simulink model "Assignment8"  (R2017a)
settings: Solver=FixedStepAuto  StartTime=0.0  StopTime=10.0  FixedStep=1e-5  RelTol=1e-3
values from neighbouring files (symbols this model uses):
  B = 0.1    [Assignment8_case1.m]    (also in Assignment8_case2.m; Assignment8_case3.m; Assignment8_case4.m; Assignment8_case5.m)
  FV = 10    [Assignment8_case1.m]    (also in Assignment8_case2.m = 900; Assignment8_case3.m; Assignment8_case4.m; Assignment8_case5.m)
  J = 0.01    [Assignment8_case1.m]    (also in Assignment8_case2.m; Assignment8_case3.m; Assignment8_case4.m; Assignment8_case5.m)
  K = 0.1    [Assignment8_case1.m]    (also in Assignment8_case2.m; Assignment8_case3.m; Assignment8_case4.m; Assignment8_case5.m)
  La = 0.5e-3    (= 0.0005)    [Assignment8_case1.m]    (also in Assignment8_case2.m; Assignment8_case3.m; Assignment8_case4.m; Assignment8_case5.m)
  Ra = 10    [Assignment8_case1.m]    (also in Assignment8_case2.m; Assignment8_case3.m; Assignment8_case4.m; Assignment8_case5.m)
  Step = 0    [Assignment8_case1.m]    (also in Assignment8_case2.m; Assignment8_case3.m; Assignment8_case4.m; Assignment8_case5.m)
settings Model: Creator=jms2299  LastModifiedBy=jms2299

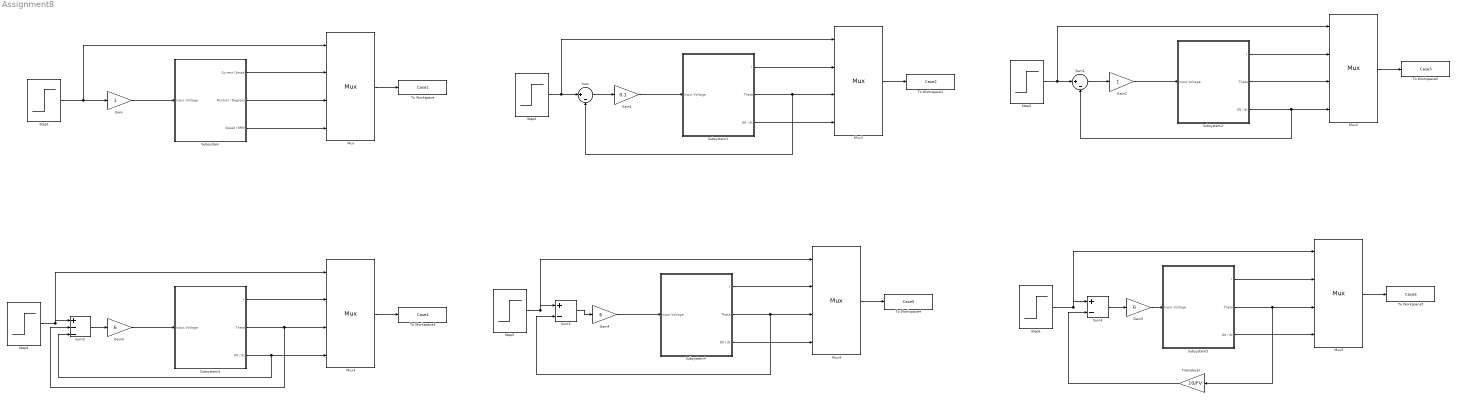
== system Assignment8 ==
  Gain : Gain
  Gain1 : Gain  Gain=0.1
  Gain2 : Gain
  Gain3 : Gain  Gain=6
  Gain4 : Gain  Gain=6
  Gain5 : Gain  Gain=6
  Mux{,1..5} (6 alike) : Mux
  Step{1..6} (6 alike) : Step  Time=Step  After=FV  SampleTime=0
  Subsystem : Subsystem
  Subsystem1 : Subsystem
  Subsystem2 : Subsystem
  Subsystem3 : Subsystem
  Subsystem4 : Subsystem
  Subsystem5 : Subsystem
  Sum{,1,3..4} (4 alike) : Sum  Inputs=|+-
  Sum2 : Sum  Inputs=|+--
  To Workspace : ToWorkspace  VariableName=Case1  SampleTime=-1
  To Workspace1 : ToWorkspace  VariableName=Case2  SampleTime=-1
  To Workspace2 : ToWorkspace  VariableName=Case3  SampleTime=-1
  To Workspace3 : ToWorkspace  VariableName=Case4  SampleTime=-1
  To Workspace4 : ToWorkspace  VariableName=Case5  SampleTime=-1
  To Workspace5 : ToWorkspace  VariableName=Case6  SampleTime=-1
  Transducer : Gain  Gain=10/FV
  wires:
  Step1/1 -> Mux/1, Gain/1
  Subsystem/2(Position (Degrees)) -> Mux/3
  Subsystem/1(Current (Amps)) -> Mux/2
  Subsystem/3(Speed (RPM)) -> Mux/4
  Mux/1 -> To Workspace/1
  Gain/1 -> Subsystem/1(Input Voltage)
  Mux1/1 -> To Workspace1/1
  Gain1/1 -> Subsystem1/1(Input Voltage)
  Subsystem1/3(D0 / dt) -> Mux1/4
  Subsystem1/1(I) -> Mux1/2
  Sum/1 -> Gain1/1
  Step2/1 -> Mux1/1, Sum/1
  Subsystem1/2(Theta) -> Sum/2, Mux1/3
  Step3/1 -> Mux2/1, Sum1/1
  Subsystem2/3(D0 / dt) -> Sum1/2, Mux2/4
  Subsystem2/2(Theta) -> Mux2/3
  Subsystem2/1(I) -> Mux2/2
  Gain2/1 -> Subsystem2/1(Input Voltage)
  Sum1/1 -> Gain2/1
  Mux2/1 -> To Workspace2/1
  Step4/1 -> Mux3/1, Sum2/1
  Subsystem3/3(D0 / dt) -> Sum2/3, Mux3/4
  Subsystem3/2(Theta) -> Sum2/2, Mux3/3
  Subsystem3/1(I) -> Mux3/2
  Gain3/1 -> Subsystem3/1(Input Voltage)
  Sum2/1 -> Gain3/1
  Mux3/1 -> To Workspace3/1
  Mux4/1 -> To Workspace4/1
  Subsystem4/2(Theta) -> Sum3/2, Mux4/3
  Subsystem4/1(I) -> Mux4/2
  Step5/1 -> Mux4/1, Sum3/1
  Subsystem4/3(D0 / dt) -> Mux4/4
  Sum3/1 -> Gain4/1
  Gain4/1 -> Subsystem4/1(Input Voltage)
  Subsystem5/3(D0 / dt) -> Mux5/4
  Subsystem5/2(Theta) -> Transducer/1, Mux5/3
  Subsystem5/1(I) -> Mux5/2
  Mux5/1 -> To Workspace5/1
  Transducer/1 -> Sum4/2
  Step6/1 -> Mux5/1, Sum4/1
  Sum4/1 -> Gain5/1
  Gain5/1 -> Subsystem5/1(Input Voltage)

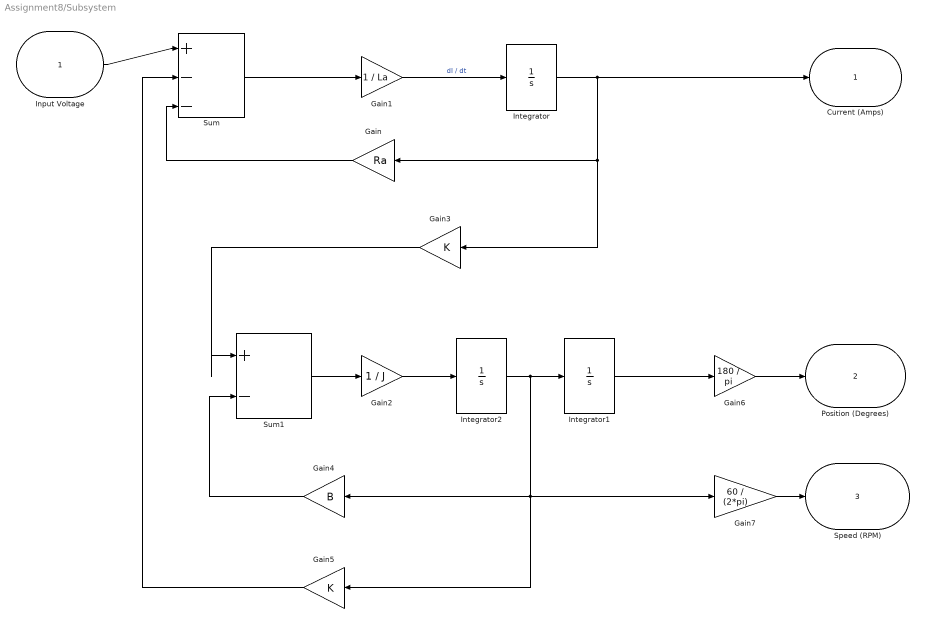
== system Assignment8/Subsystem ==
  Input Voltage : Inport
  Gain : Gain  Gain=Ra
  Gain1 : Gain  Gain=1 / La
  Gain2 : Gain  Gain=1 / J
  Gain3 : Gain  Gain=K
  Gain4 : Gain  Gain=B
  Gain5 : Gain  Gain=K
  Gain6 : Gain  Gain=180 / pi
  Gain7 : Gain  Gain=60 / (2*pi)
  Integrator : Integrator
  Integrator1 : Integrator
  Integrator2 : Integrator
  Sum : Sum  Inputs=|+--
  Sum1 : Sum  Inputs=|+-
  Current (Amps) : Outport
  Position (Degrees) : Outport  Port=2
  Speed (RPM) : Outport  Port=3
  wires:
  Sum1/1 -> Gain2/1
  Integrator/1 -> Current (Amps)/1, Gain3/1, Gain/1
  Gain3/1 -> Sum1/1
  Gain/1 -> Sum/3
  Gain1/1 -> Integrator/1  "dI / dt"
  Gain2/1 -> Integrator2/1
  Sum/1 -> Gain1/1
  Gain4/1 -> Sum1/2
  Gain5/1 -> Sum/2
  Integrator2/1 -> Gain7/1, Gain4/1, Gain5/1, Integrator1/1
  Input Voltage/1 -> Sum/1
  Integrator1/1 -> Gain6/1
  Gain6/1 -> Position (Degrees)/1
  Gain7/1 -> Speed (RPM)/1

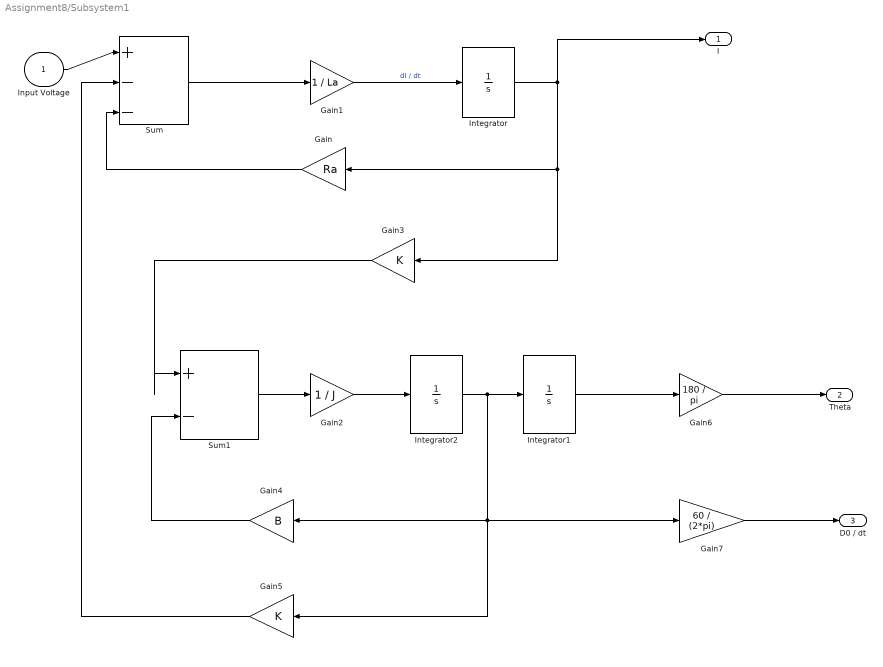
== system Assignment8/Subsystem1 ==
  Input Voltage : Inport
  Gain : Gain  Gain=Ra
  Gain1 : Gain  Gain=1 / La
  Gain2 : Gain  Gain=1 / J
  Gain3 : Gain  Gain=K
  Gain4 : Gain  Gain=B
  Gain5 : Gain  Gain=K
  Gain6 : Gain  Gain=180 / pi
  Gain7 : Gain  Gain=60 / (2*pi)
  Integrator : Integrator
  Integrator1 : Integrator
  Integrator2 : Integrator
  Sum : Sum  Inputs=|+--
  Sum1 : Sum  Inputs=|+-
  I : Outport
  Theta : Outport  Port=2
  D0 / dt : Outport  Port=3
  wires:
  Sum1/1 -> Gain2/1
  Integrator/1 -> I/1, Gain3/1, Gain/1
  Gain3/1 -> Sum1/1
  Gain/1 -> Sum/3
  Gain1/1 -> Integrator/1  "dI / dt"
  Gain2/1 -> Integrator2/1
  Sum/1 -> Gain1/1
  Gain4/1 -> Sum1/2
  Gain5/1 -> Sum/2
  Integrator2/1 -> Gain7/1, Gain4/1, Gain5/1, Integrator1/1
  Input Voltage/1 -> Sum/1
  Integrator1/1 -> Gain6/1
  Gain6/1 -> Theta/1
  Gain7/1 -> D0 / dt/1

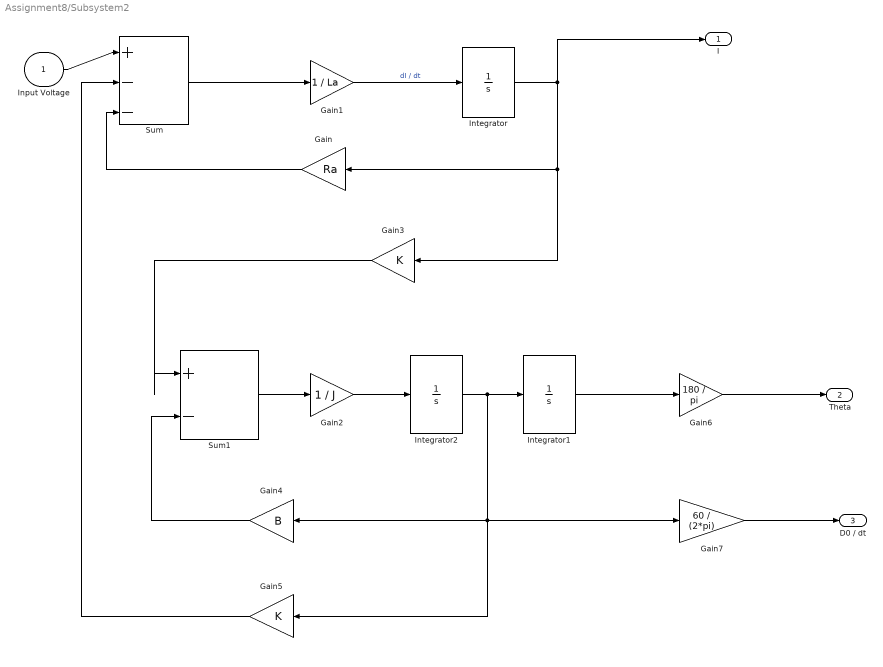
== system Assignment8/Subsystem2 ==
  Input Voltage : Inport
  Gain : Gain  Gain=Ra
  Gain1 : Gain  Gain=1 / La
  Gain2 : Gain  Gain=1 / J
  Gain3 : Gain  Gain=K
  Gain4 : Gain  Gain=B
  Gain5 : Gain  Gain=K
  Gain6 : Gain  Gain=180 / pi
  Gain7 : Gain  Gain=60 / (2*pi)
  Integrator : Integrator
  Integrator1 : Integrator
  Integrator2 : Integrator
  Sum : Sum  Inputs=|+--
  Sum1 : Sum  Inputs=|+-
  I : Outport
  Theta : Outport  Port=2
  D0 / dt : Outport  Port=3
  wires:
  Sum1/1 -> Gain2/1
  Integrator/1 -> I/1, Gain3/1, Gain/1
  Gain3/1 -> Sum1/1
  Gain/1 -> Sum/3
  Gain1/1 -> Integrator/1  "dI / dt"
  Gain2/1 -> Integrator2/1
  Sum/1 -> Gain1/1
  Gain4/1 -> Sum1/2
  Gain5/1 -> Sum/2
  Integrator2/1 -> Gain7/1, Gain4/1, Gain5/1, Integrator1/1
  Input Voltage/1 -> Sum/1
  Integrator1/1 -> Gain6/1
  Gain6/1 -> Theta/1
  Gain7/1 -> D0 / dt/1

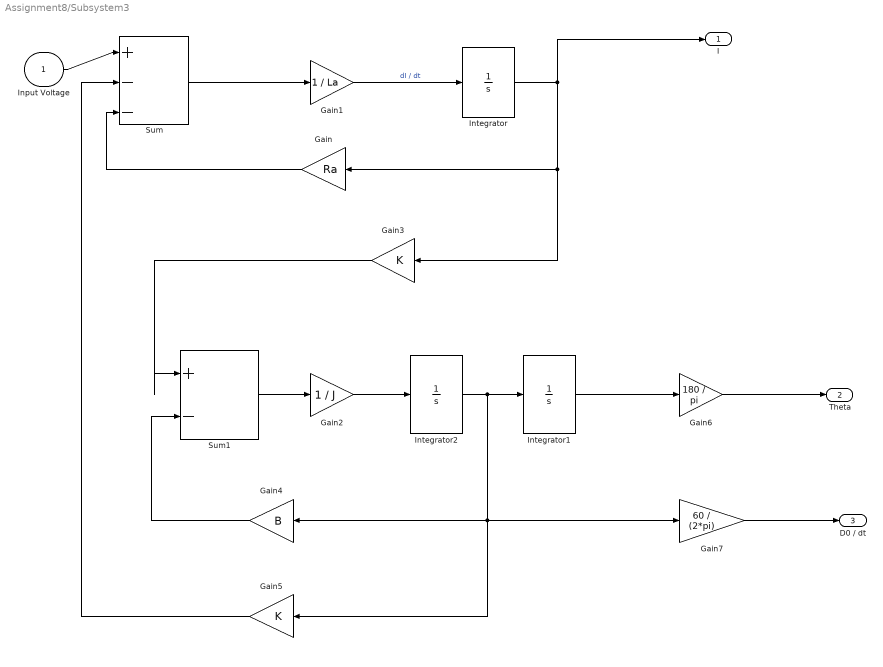
== system Assignment8/Subsystem3 ==
  Input Voltage : Inport
  Gain : Gain  Gain=Ra
  Gain1 : Gain  Gain=1 / La
  Gain2 : Gain  Gain=1 / J
  Gain3 : Gain  Gain=K
  Gain4 : Gain  Gain=B
  Gain5 : Gain  Gain=K
  Gain6 : Gain  Gain=180 / pi
  Gain7 : Gain  Gain=60 / (2*pi)
  Integrator : Integrator
  Integrator1 : Integrator
  Integrator2 : Integrator
  Sum : Sum  Inputs=|+--
  Sum1 : Sum  Inputs=|+-
  I : Outport
  Theta : Outport  Port=2
  D0 / dt : Outport  Port=3
  wires:
  Sum1/1 -> Gain2/1
  Integrator/1 -> I/1, Gain3/1, Gain/1
  Gain3/1 -> Sum1/1
  Gain/1 -> Sum/3
  Gain1/1 -> Integrator/1  "dI / dt"
  Gain2/1 -> Integrator2/1
  Sum/1 -> Gain1/1
  Gain4/1 -> Sum1/2
  Gain5/1 -> Sum/2
  Integrator2/1 -> Gain7/1, Gain4/1, Gain5/1, Integrator1/1
  Input Voltage/1 -> Sum/1
  Integrator1/1 -> Gain6/1
  Gain6/1 -> Theta/1
  Gain7/1 -> D0 / dt/1

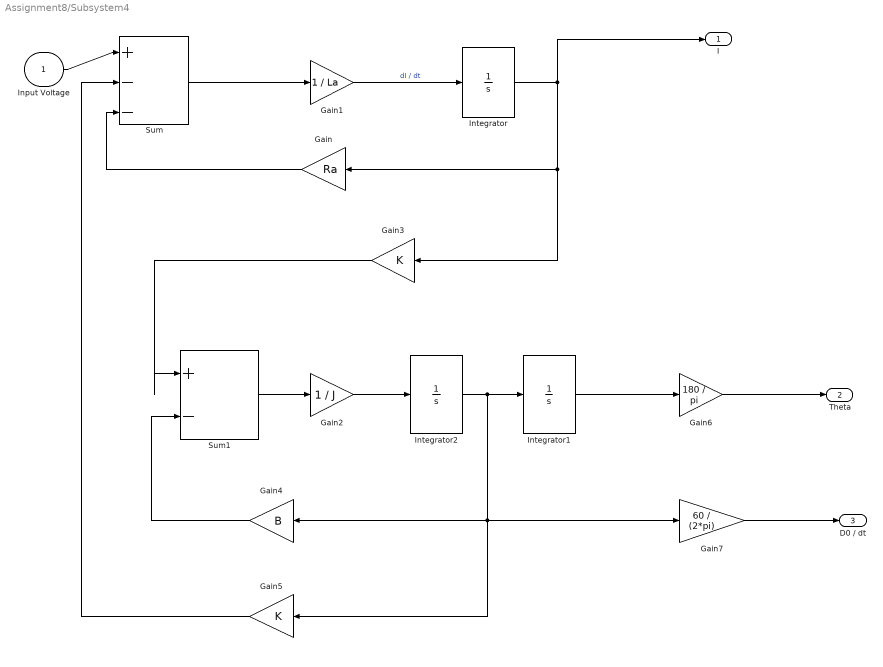
== system Assignment8/Subsystem4 ==
  Input Voltage : Inport
  Gain : Gain  Gain=Ra
  Gain1 : Gain  Gain=1 / La
  Gain2 : Gain  Gain=1 / J
  Gain3 : Gain  Gain=K
  Gain4 : Gain  Gain=B
  Gain5 : Gain  Gain=K
  Gain6 : Gain  Gain=180 / pi
  Gain7 : Gain  Gain=60 / (2*pi)
  Integrator : Integrator
  Integrator1 : Integrator
  Integrator2 : Integrator
  Sum : Sum  Inputs=|+--
  Sum1 : Sum  Inputs=|+-
  I : Outport
  Theta : Outport  Port=2
  D0 / dt : Outport  Port=3
  wires:
  Sum1/1 -> Gain2/1
  Integrator/1 -> I/1, Gain3/1, Gain/1
  Gain3/1 -> Sum1/1
  Gain/1 -> Sum/3
  Gain1/1 -> Integrator/1  "dI / dt"
  Gain2/1 -> Integrator2/1
  Sum/1 -> Gain1/1
  Gain4/1 -> Sum1/2
  Gain5/1 -> Sum/2
  Integrator2/1 -> Gain7/1, Gain4/1, Gain5/1, Integrator1/1
  Input Voltage/1 -> Sum/1
  Integrator1/1 -> Gain6/1
  Gain6/1 -> Theta/1
  Gain7/1 -> D0 / dt/1

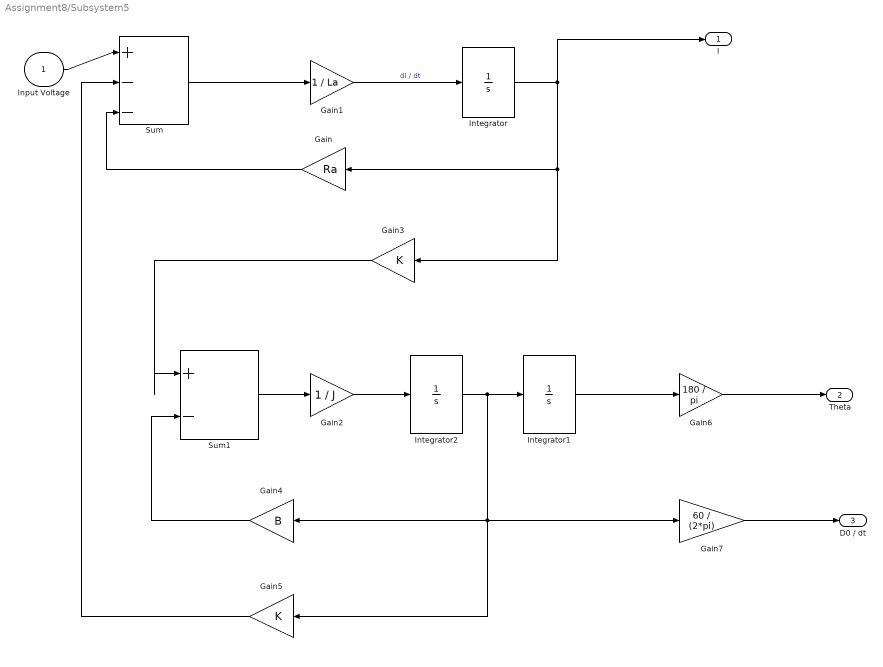
== system Assignment8/Subsystem5 ==
  Input Voltage : Inport
  Gain : Gain  Gain=Ra
  Gain1 : Gain  Gain=1 / La
  Gain2 : Gain  Gain=1 / J
  Gain3 : Gain  Gain=K
  Gain4 : Gain  Gain=B
  Gain5 : Gain  Gain=K
  Gain6 : Gain  Gain=180 / pi
  Gain7 : Gain  Gain=60 / (2*pi)
  Integrator : Integrator
  Integrator1 : Integrator
  Integrator2 : Integrator
  Sum : Sum  Inputs=|+--
  Sum1 : Sum  Inputs=|+-
  I : Outport
  Theta : Outport  Port=2
  D0 / dt : Outport  Port=3
  wires:
  Sum1/1 -> Gain2/1
  Integrator/1 -> I/1, Gain3/1, Gain/1
  Gain3/1 -> Sum1/1
  Gain/1 -> Sum/3
  Gain1/1 -> Integrator/1  "dI / dt"
  Gain2/1 -> Integrator2/1
  Sum/1 -> Gain1/1
  Gain4/1 -> Sum1/2
  Gain5/1 -> Sum/2
  Integrator2/1 -> Gain7/1, Gain4/1, Gain5/1, Integrator1/1
  Input Voltage/1 -> Sum/1
  Integrator1/1 -> Gain6/1
  Gain6/1 -> Theta/1
  Gain7/1 -> D0 / dt/1
